simulink model "Kart"  (Simulink 8.6)
settings: Solver=ode45  StartTime=0.0  StopTime=40  RelTol=1e-3
values from neighbouring files (symbols this model uses):
  AD = 0.5*A*Cd*p    (= 0.1803)    [Ninad_deshpande_Kartdata.m]
  FD = Mass*g*RRc    (= 29.43)    [Ninad_deshpande_Kartdata.m]
  Gr = 2    [Ninad_deshpande_Kartdata.m]
  KT = 0.12    [Ninad_deshpande_Kartdata.m]
  KV = 0.127    [Ninad_deshpande_Kartdata.m]
  La = 0.01    [Ninad_deshpande_Kartdata.m]
  Mass = 150    [Ninad_deshpande_Kartdata.m]
  Ra = 0.053    [Ninad_deshpande_Kartdata.m]
  Rw = .10    (= 0.1)    [Ninad_deshpande_Kartdata.m]
undefined symbols (not defined in the file or in its folder): vt, xt
libraries: simulink x1
settings Model: Creator=Bob  LastModifiedBy=pc
settings SolverCC: ZeroCrossControl=DisableAll
settings DataIOCC: LimitDataPoints=off  SaveFormat=StructureWithTime
settings DebuggingCC: FcnCallInpInsideContextMsg=UseLocalSettings

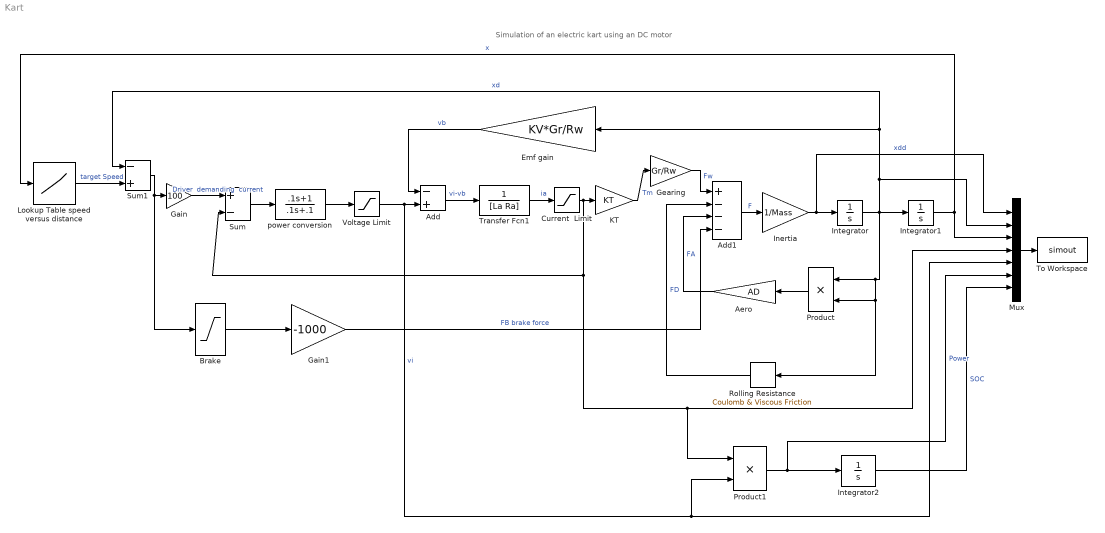
== system Kart ==
  note: Simulation of an electric kart using an DC motor
  Add : Sum  Inputs=-+
  Add1 : Sum  Inputs=+---
  Aero : Gain  Gain=AD
  Brake : Saturate  UpperLimit=0  LowerLimit=-1000
  Current  Limit : Saturate  UpperLimit=300  LowerLimit=0
  Emf gain : Gain  Gain=KV*Gr/Rw
  Gain : Gain  Gain=100
  Gain1 : Gain  Gain=-1000
  Gearing : Gain  Gain=Gr/Rw
  Inertia : Gain  Gain=1/Mass
  Integrator : Integrator
  Integrator1 : Integrator
  Integrator2 : Integrator
  KT : Gain  Gain=KT
  Lookup Table speed versus distance : Lookup  InputValues=xt  Table=vt
  Mux : Mux  Inputs=7
  Product : Product  RndMeth=Zero
  Product1 : Product  RndMeth=Zero
  Rolling Resistance : simulink/Discontinuities/Coulomb & Viscous Friction  offset=[FD]  gain=0
  Sum : Sum  Inputs=+-
  Sum1 : Sum  Inputs=-+
  To Workspace : ToWorkspace  VariableName=simout  SaveFormat=Structure  SampleTime=-1
  Transfer Fcn1 : TransferFcn  Denominator=[La Ra]
  Voltage Limit : Saturate  UpperLimit=48  LowerLimit=0
  power conversion : TransferFcn  Numerator=[.1 1]  Denominator=[.1 .1]
  wires:
  Add1/1 -> Inertia/1  "F"
  Gearing/1 -> Add1/1  "Fw"
  Add/1 -> Transfer Fcn1/1  "vi-vb"
  Emf gain/1 -> Add/1  "vb"
  Product/1 -> Aero/1
  Aero/1 -> Add1/3  "FA"
  Integrator/1 -> Mux/2, Emf gain/1, Sum1/1, Product/1, Product/2, Rolling Resistance/1, Integrator1/1  "xd"
  Integrator1/1 -> Mux/3, Lookup Table speed versus distance/1  "x"
  Mux/1 -> To Workspace/1
  Voltage Limit/1 -> Add/2, Mux/5, Product1/2  "vi"
  Product1/1 -> Integrator2/1, Mux/6  "Power"
  power conversion/1 -> Voltage Limit/1
  Integrator2/1 -> Mux/7  "SOC"
  Sum/1 -> power conversion/1
  Lookup Table speed versus distance/1 -> Sum1/2  "target Speed"
  Gain/1 -> Sum/1  "Driver  demanding  current"
  Sum1/1 -> Gain/1, Brake/1
  Transfer Fcn1/1 -> Current  Limit/1  "ia"
  Current  Limit/1 -> Sum/2, Mux/4, Product1/1, KT/1
  KT/1 -> Gearing/1  "Tm"
  Inertia/1 -> Integrator/1, Mux/1  "xdd"
  Brake/1 -> Gain1/1
  Gain1/1 -> Add1/4  "FB brake force"
  Rolling Resistance/1 -> Add1/2  "FD"
